simulink model "ES205_lab_5_upper_model_orig"  (R2021a)
settings: Solver=VariableStepAuto  StartTime=0.0  StopTime=tf_upper  MaxStep=maxstep  RelTol=tol  AbsTol=tol
values from neighbouring files (symbols this model uses):
  a1 = 3.49    [ES205_lab_5_script.m]
  Aout1 = pi * (d1/2)^2    (= 0.0881413088873)    [ES205_lab_5_script.m]
  Atank1 = 22.94    [ES205_lab_5_script.m]
  b2 = 0.5    [ES205_lab_5_script.m]
  Cd1_orig = 0.7    [ES205_lab_5_script.m]
  g = 32.2 * 12    (= 386.4)    [ES205_lab_5_script.m]
  h1_0_single = h1data_single(1)    [ES205_lab_5_script.m]
settings Model: Creator=schimmer  LastModifiedBy=schimmer
settings DataIOCC: SaveOutput=off  SignalLogging=off  DSMLogging=off  SaveTime=off  ReturnWorkspaceOutputs=off  OutputOption=SpecifiedOutputTimes  OutputTimes=tdata_upper

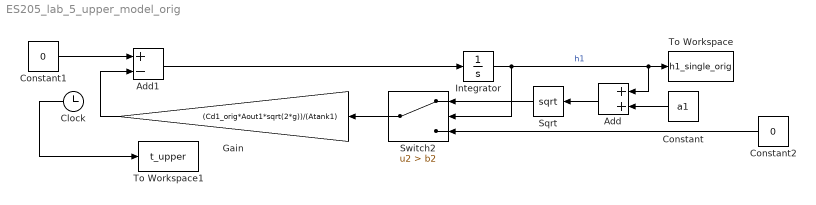
== system ES205_lab_5_upper_model_orig ==
  Add : Sum
  Add1 : Sum  Inputs=+-
  Clock : Clock
  Constant : Constant  Value=a1
  Constant1 : Constant  Value=0
  Constant2 : Constant  Value=0
  Gain : Gain  Gain=(Cd1_orig*Aout1*sqrt(2*g))/(Atank1)
  Integrator : Integrator  InitialCondition=h1_0_single
  Sqrt : Sqrt  SaturateOnIntegerOverflow=on
  Switch2 : Switch  Criteria=u2 > Threshold  Threshold=b2
  To Workspace : ToWorkspace  VariableName=h1_single_orig  SampleTime=-1
  To Workspace1 : ToWorkspace  VariableName=t_upper  SampleTime=-1
  wires:
  Clock/1 -> To Workspace1/1
  Integrator/1 -> Add/1, To Workspace/1, Switch2/2  "h1"
  Sqrt/1 -> Switch2/1
  Add/1 -> Sqrt/1
  Constant/1 -> Add/2
  Switch2/1 -> Gain/1
  Constant2/1 -> Switch2/3
  Add1/1 -> Integrator/1
  Gain/1 -> Add1/2
  Constant1/1 -> Add1/1
